simulink model "p102"  (R2015a)
settings: Solver=ode3  StartTime=0.0  StopTime=simtime  FixedStep=step  RelTol=1e-3
values from neighbouring files (symbols this model uses):
  a = (M*L)/2+m*l    (= 0.03371)    [lab3.m]
  beta = 0.01    [lab3.m]
  dteta0 = 0    [lab3.m]
  g = 9.8    [lab3.m]
  J = (1/3)*M*(L^2)+m*(l^2)    (= 0.00422554333333)    [lab3.m]
  k = 0.35    [lab3.m]
  teta0 = pi/4    (= 0.785398163397)    [lab3.m]
settings Model: Creator=Pedro  LastModifiedBy=Pedro

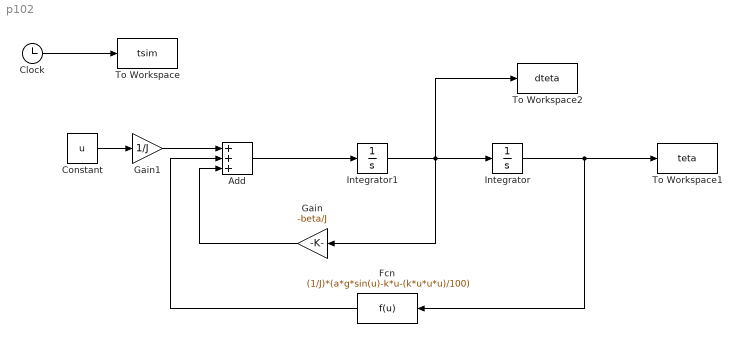
== system p102 ==
  Add : Sum  Inputs=+++
  Clock : Clock
  Constant : Constant  Value=u
  Fcn : Fcn  Expr=(1/J)*(a*g*sin(u)-k*u-(k*u*u*u)/100)
  Gain : Gain  Gain=-beta/J
  Gain1 : Gain  Gain=1/J
  Integrator : Integrator  InitialCondition=teta0
  Integrator1 : Integrator  InitialCondition=dteta0
  To Workspace : ToWorkspace  VariableName=tsim  SampleTime=-1
  To Workspace1 : ToWorkspace  VariableName=teta  SampleTime=-1
  To Workspace2 : ToWorkspace  VariableName=dteta  SampleTime=-1
  wires:
  Clock/1 -> To Workspace/1
  Integrator/1 -> Fcn/1, To Workspace1/1
  Integrator1/1 -> To Workspace2/1, Gain/1, Integrator/1
  Add/1 -> Integrator1/1
  Gain/1 -> Add/3
  Fcn/1 -> Add/2
  Constant/1 -> Gain1/1
  Gain1/1 -> Add/1
